simulink model "Observer_mode_model9"  (R2024b)
settings: Solver=FixedStepAuto  StartTime=0.0  StopTime=10.0  FixedStep=0.01  RelTol=1e-3
settings Model: Creator=The MathWorks, Inc.  LastModifiedBy=arena
settings SolverCC: MaxZcPerStep=1
settings DataIOCC: SaveFormat=Array  SignalLogging=off  DSMLogging=off
settings OptimizationCC: ReuseModelBlockBuffer=off
settings DebuggingCC: UnconnectedInputMsg=warning  UnconnectedOutputMsg=warning  UnconnectedLineMsg=warning
settings ModelReferenceCC: EnableRefExpFcnMdlSchedulingChecks=on
settings RTWCC: GPUComputeCapability=3.5  DLArmComputeVersion=19.05
settings ConfigComp: DVTestSuiteOptimization=Auto  DVDefectChecker=off  DVDetectOutOfBounds=on  DVModelReferenceHarness=on  DVHarnessSource=Signal Editor

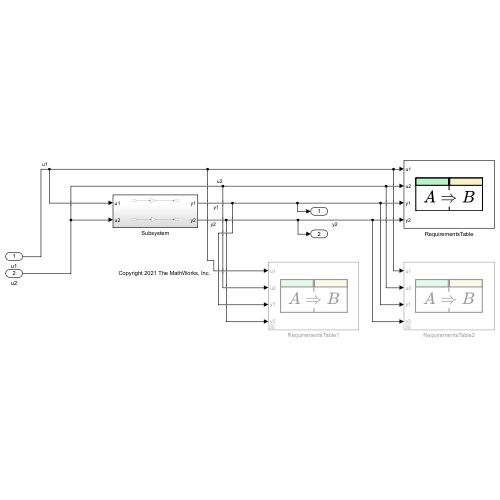
[thumbnail: Simulink's stored preview of the top-level diagram]
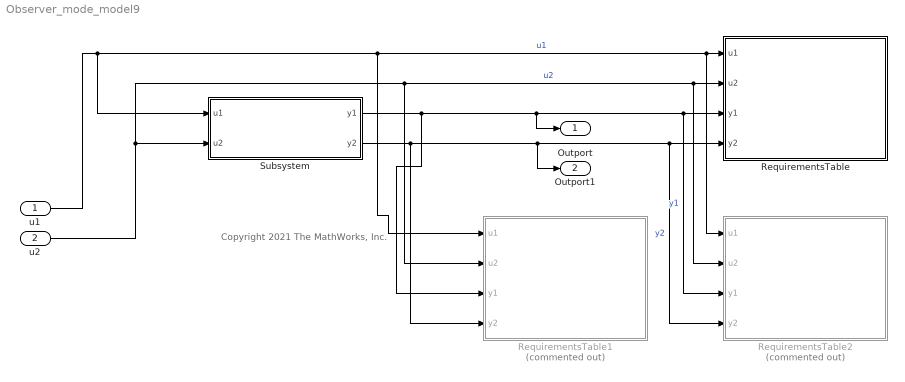
== system Observer_mode_model9 ==
  note: Copyright 2021 The MathWorks, Inc.
  u1 : Inport
  u2 : Inport  Port=2
  RequirementsTable : Requirements Table  TreatAsAtomicUnit=on
  RequirementsTable1 : Requirements Table  Commented=on  TreatAsAtomicUnit=on
  RequirementsTable2 : Requirements Table  Commented=on  TreatAsAtomicUnit=on
  Subsystem : Subsystem
  Outport : Outport
  Outport1 : Outport  Port=2
  wires:
  Subsystem/2(y2) -> RequirementsTable1/4(y2), Outport1/1, RequirementsTable/4(y2), RequirementsTable2/4(y2)  "y2"
  u1/1 -> RequirementsTable/1(u1), RequirementsTable2/1(u1), RequirementsTable1/1(u1), Subsystem/1(u1)  "u1"
  u2/1 -> RequirementsTable/2(u2), RequirementsTable2/2(u2), RequirementsTable1/2(u2), Subsystem/2(u2)  "u2"
  Subsystem/1(y1) -> RequirementsTable1/3(y1), Outport/1, RequirementsTable/3(y1), RequirementsTable2/3(y1)  "y1"

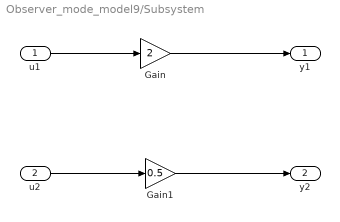
== system Observer_mode_model9/Subsystem ==
  u1 : Inport
  u2 : Inport  Port=2
  Gain : Gain  Gain=2
  Gain1 : Gain  Gain=0.5
  y1 : Outport
  y2 : Outport  Port=2
  wires:
  u1/1 -> Gain/1
  u2/1 -> Gain1/1
  Gain1/1 -> y2/1
  Gain/1 -> y1/1

== stateflow chart Observer_mode_model9/RequirementsTable1 ==
  (default) -> (junction 1073742902)
  (junction 1073742902) -> (junction 1073742903) : {
      | % SF_REQ_REV_07
      | }
  (junction 1073742903) -> (junction 1073742905) : {
      | % ExcEvals:
      | % PriEvals:
      | }
  (junction 1073742905) -> (junction 1073742907) : {
      | % HEADER_ASSIGNMENTS
      |
      | }
  (junction 1073742907) -> (junction 1073742909) : {
      | % START_A_4
      | }
  (junction 1073742909) -> (junction 1073742911) : {
      | }
  (junction 1073742911) -> (junction 1073742913)
  (junction 1073742913) -> (junction 1073742915) : {
      | }
  (junction 1073742915) -> (junction 1073742917) : {
      | % END_A_4
      | }
  (junction 1073742917) -> (junction 1073742919) : {
      | % START_R_7
      | }
  (junction 1073742919) -> (junction 1073742921) : {
      | }
  (junction 1073742921) -> (junction 1073742923)
  (junction 1073742923) -> (junction 1073742925) [order 1] : [(u1 > 0)]
  (junction 1073742923) -> (junction 1073742931) [order 2]
  (junction 1073742925) -> (junction 1073742927) : {
      | reqtable_postcondition((y1 > - 0.5), 'R:1');
      |
      |
      | }
  (junction 1073742927) -> (junction 1073742929) : {
      | }
  (junction 1073742929) -> (junction 1073742931)
  (junction 1073742931) -> (junction 1073742933)
  (junction 1073742933) -> (junction 1073742935) : {
      | % END_R_7
      | }
  (junction 1073742935) -> (junction 1073742937) : {
      | % START_R_1
      | }
  (junction 1073742937) -> (junction 1073742939) : {
      | }
  (junction 1073742939) -> (junction 1073742941)
  (junction 1073742941) -> (junction 1073742943) [order 1] : [(u2 > 0)]
  (junction 1073742941) -> (junction 1073742949) [order 2]
  (junction 1073742943) -> (junction 1073742945) : {
      | reqtable_postcondition((y2 > - 0.5), 'R:2');
      |
      |
      | }
  (junction 1073742945) -> (junction 1073742947) : {
      | }
  (junction 1073742947) -> (junction 1073742949)
  (junction 1073742949) -> (junction 1073742951)
  (junction 1073742951) -> (junction 1073742953) : {
      | % END_R_1
      | }
  (junction 1073742953) -> (junction 1073742955) : {
      | % START_R_10
      | }
  (junction 1073742955) -> (junction 1073742957) : {
      | }
  (junction 1073742957) -> (junction 1073742959) : {
      | reqtable_postcondition((0 < y1 || 0 >= y1 || 0 < y2 || 0 >= y2), 'R:3');
      |
      |
      | }
  (junction 1073742959) -> (junction 1073742961) : {
      | }
  (junction 1073742961) -> (junction 1073742963) : {
      | % END_R_10
      | }
  data: u1 input; u2 input; y1 input; y2 input

== stateflow chart Observer_mode_model9/RequirementsTable2 ==
  (default) -> (junction 1073742902)
  (junction 1073742902) -> (junction 1073742903) : {
      | % SF_REQ_REV_07
      | }
  (junction 1073742903) -> (junction 1073742905) : {
      | % ExcEvals:
      | % PriEvals:
      | }
  (junction 1073742905) -> (junction 1073742907) : {
      | % HEADER_ASSIGNMENTS
      |
      | }
  (junction 1073742907) -> (junction 1073742909) : {
      | % START_A_4
      | }
  (junction 1073742909) -> (junction 1073742911) : {
      | }
  (junction 1073742911) -> (junction 1073742913)
  (junction 1073742913) -> (junction 1073742915) : {
      | }
  (junction 1073742915) -> (junction 1073742917) : {
      | % END_A_4
      | }
  (junction 1073742917) -> (junction 1073742919) : {
      | % START_R_7
      | }
  (junction 1073742919) -> (junction 1073742921) : {
      | }
  (junction 1073742921) -> (junction 1073742923)
  (junction 1073742923) -> (junction 1073742925) [order 1] : [(u1 > - 0.5)]
  (junction 1073742923) -> (junction 1073742931) [order 2]
  (junction 1073742925) -> (junction 1073742927) : {
      | reqtable_postcondition((y1 > 0), 'R:1');
      |
      |
      | }
  (junction 1073742927) -> (junction 1073742929) : {
      | }
  (junction 1073742929) -> (junction 1073742931)
  (junction 1073742931) -> (junction 1073742933)
  (junction 1073742933) -> (junction 1073742935) : {
      | % END_R_7
      | }
  (junction 1073742935) -> (junction 1073742937) : {
      | % START_R_1
      | }
  (junction 1073742937) -> (junction 1073742939) : {
      | }
  (junction 1073742939) -> (junction 1073742941)
  (junction 1073742941) -> (junction 1073742943) [order 1] : [(u2 > - 0.5)]
  (junction 1073742941) -> (junction 1073742949) [order 2]
  (junction 1073742943) -> (junction 1073742945) : {
      | reqtable_postcondition((y2 > 0), 'R:2');
      |
      |
      | }
  (junction 1073742945) -> (junction 1073742947) : {
      | }
  (junction 1073742947) -> (junction 1073742949)
  (junction 1073742949) -> (junction 1073742951)
  (junction 1073742951) -> (junction 1073742953) : {
      | % END_R_1
      | }
  (junction 1073742953) -> (junction 1073742955) : {
      | % START_R_10
      | }
  (junction 1073742955) -> (junction 1073742957) : {
      | }
  (junction 1073742957) -> (junction 1073742959) : {
      | reqtable_postcondition((0 < y1 || 0 >= y1 || 0 < y2 || 0 >= y2), 'R:3');
      |
      |
      | }
  (junction 1073742959) -> (junction 1073742961) : {
      | }
  (junction 1073742961) -> (junction 1073742963) : {
      | % END_R_10
      | }
  data: u1 input; u2 input; y1 input; y2 input

== stateflow chart Observer_mode_model9/RequirementsTable ==
  (default) -> (junction 1073742902)
  (junction 1073742902) -> (junction 1073742903) : {
      | % SF_REQ_REV_07
      | }
  (junction 1073742903) -> (junction 1073742905) : {
      | % ExcEvals:
      | % PriEvals:
      | }
  (junction 1073742905) -> (junction 1073742907) : {
      | % HEADER_ASSIGNMENTS
      |
      | }
  (junction 1073742907) -> (junction 1073742909) : {
      | % START_A_4
      | }
  (junction 1073742909) -> (junction 1073742911) : {
      | }
  (junction 1073742911) -> (junction 1073742913)
  (junction 1073742913) -> (junction 1073742915) : {
      | }
  (junction 1073742915) -> (junction 1073742917) : {
      | % END_A_4
      | }
  (junction 1073742917) -> (junction 1073742919) : {
      | % START_R_7
      | }
  (junction 1073742919) -> (junction 1073742921) : {
      | }
  (junction 1073742921) -> (junction 1073742923)
  (junction 1073742923) -> (junction 1073742925) [order 1] : [(u1 > 0)]
  (junction 1073742923) -> (junction 1073742931) [order 2]
  (junction 1073742925) -> (junction 1073742927) : {
      | reqtable_postcondition((y1 > 0), 'R:1');
      |
      |
      | }
  (junction 1073742927) -> (junction 1073742929) : {
      | }
  (junction 1073742929) -> (junction 1073742931)
  (junction 1073742931) -> (junction 1073742933)
  (junction 1073742933) -> (junction 1073742935) : {
      | % END_R_7
      | }
  (junction 1073742935) -> (junction 1073742937) : {
      | % START_R_1
      | }
  (junction 1073742937) -> (junction 1073742939) : {
      | }
  (junction 1073742939) -> (junction 1073742941)
  (junction 1073742941) -> (junction 1073742943) [order 1] : [(u2 > 0)]
  (junction 1073742941) -> (junction 1073742949) [order 2]
  (junction 1073742943) -> (junction 1073742945) : {
      | reqtable_postcondition((y2 > 0), 'R:2');
      |
      |
      | }
  (junction 1073742945) -> (junction 1073742947) : {
      | }
  (junction 1073742947) -> (junction 1073742949)
  (junction 1073742949) -> (junction 1073742951)
  (junction 1073742951) -> (junction 1073742953) : {
      | % END_R_1
      | }
  (junction 1073742953) -> (junction 1073742955) : {
      | % START_R_10
      | }
  (junction 1073742955) -> (junction 1073742957) : {
      | }
  (junction 1073742957) -> (junction 1073742959) : {
      | reqtable_postcondition((0 < y1 || 0 >= y1 || 0 < y2 || 0 >= y2), 'R:3');
      |
      |
      | }
  (junction 1073742959) -> (junction 1073742961) : {
      | }
  (junction 1073742961) -> (junction 1073742963) : {
      | % END_R_10
      | }
  data: u1 input; u2 input; y1 input; y2 input
